simulink library "INT_PhyMod_CalcCor"  (R2016b)
settings: Solver=VariableStepAuto  StartTime=0.0  StopTime=10.0  RelTol=1e-3
settings Model: Creator=Administrator  LastModifiedBy=Administrator

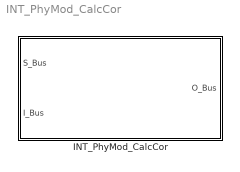
== system INT_PhyMod_CalcCor ==
  INT_PhyMod_CalcCor : Subsystem

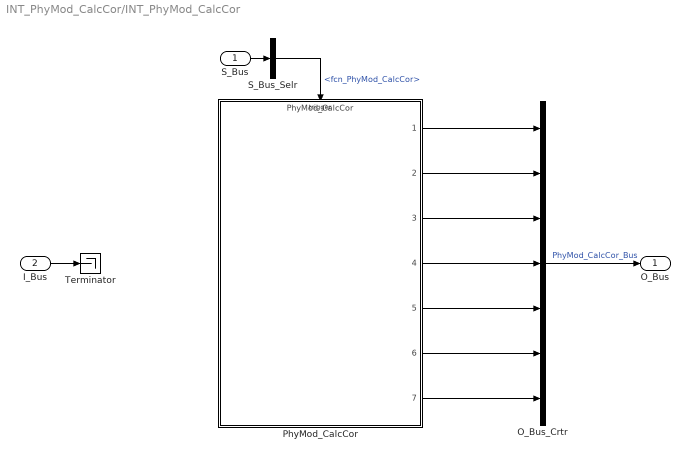
== system INT_PhyMod_CalcCor/INT_PhyMod_CalcCor ==
  S_Bus : Inport
  I_Bus : Inport  Port=2
  O_Bus_Crtr : BusCreator  Inputs=7
  PhyMod_CalcCor : ModelReference  ModelNameDialog=PhyMod_CalcCor  SimulationMode=Normal  ModelReferenceVersion=1.4  TriggerPortName=function  TriggerPortTriggerType=function-call  TriggerPortStatesWhenEnabling=held
  S_Bus_Selr : BusSelector  OutputSignals=fcn_PhyMod_CalcCor
  Terminator : Terminator
  O_Bus : Outport
  wires:
  S_Bus_Selr/1 -> PhyMod_CalcCor/Trigger  "<fcn_PhyMod_CalcCor>"
  S_Bus/1 -> S_Bus_Selr/1
  I_Bus/1 -> Terminator/1
  O_Bus_Crtr/1 -> O_Bus/1  "PhyMod_CalcCor_Bus"
  PhyMod_CalcCor/1 -> O_Bus_Crtr/1
  PhyMod_CalcCor/2 -> O_Bus_Crtr/2
  PhyMod_CalcCor/3 -> O_Bus_Crtr/3
  PhyMod_CalcCor/4 -> O_Bus_Crtr/4
  PhyMod_CalcCor/5 -> O_Bus_Crtr/5
  PhyMod_CalcCor/6 -> O_Bus_Crtr/6
  PhyMod_CalcCor/7 -> O_Bus_Crtr/7
